simulink model "untitled"  (R2021a)
settings: Solver=FixedStepDiscrete  StartTime=0.0  StopTime=inf  FixedStep=0.1  RelTol=1e-3
settings Model: SILPILModeSetting=veronly  EnablePacing=on  ExtModeTrigDuration=2  Creator=smrh1  LastModifiedBy=Abbas
settings SolverCC: AlgebraicLoopSolver=TrustRegion  AutoInsertRateTranBlk=on
settings OptimizationCC: EnhancedBackFolding=on  PassReuseOutputArgsAs=Individual arguments  ZeroExternalMemoryAtStartup=off  ZeroInternalMemoryAtStartup=off  MaxStackSize=64  OptimizeBlockOrder=speed  DifferentSizesBufferReuse=on  OptimizationCustomize=off  EfficientTunableParamExpr=on
settings DebuggingCC: ParameterTunabilityLossMsg=error  SFUnexpectedBacktrackingDiag=warning  SFNoUnconditionalDefaultTransitionDiag=warning  SFExecutionAtInitializationDiag=none  ArithmeticOperatorsInVariantConditions=warning
settings HardwareCC: ProdBitPerInt=16  ProdBitPerPointer=16  ProdBitPerSizeT=16  ProdBitPerPtrDiffT=16  ProdLargestAtomicFloat=None  ProdWordSize=8  ProdHWDeviceType=Atmel->AVR
settings SFSimCC: SimUseLocalCustomCode=off  MATLABDynamicMemAlloc=off  CustomCodeUndefinedFunction=UseInterfaceOnly
settings RTWCC: SystemTargetFile=ert.tlc  HardwareBoard=Arduino Uno  TemplateMakefile=ert_default_tmf  RTWUseLocalCustomCode=off  Toolchain=Arduino AVR  BuildConfiguration=Faster Runs
settings CodeAppCC: ForceParamTrailComments=on  IgnoreCustomStorageClasses=off  OperatorAnnotations=on  SimulinkDataObjDesc=on  SFDataObjDesc=on  InsertBlockDesc=on
settings ERTTargetCC: SupportContinuousTime=on  SupportVariableSizeSignals=on  ExtModeStaticAllocSize=250
settings ConfigComp: CovMetricSettings=dw  CovSaveCumulativeToWorkspaceVar=on  CovSaveSingleToWorkspaceVar=on  CovExternalEMLEnable=off

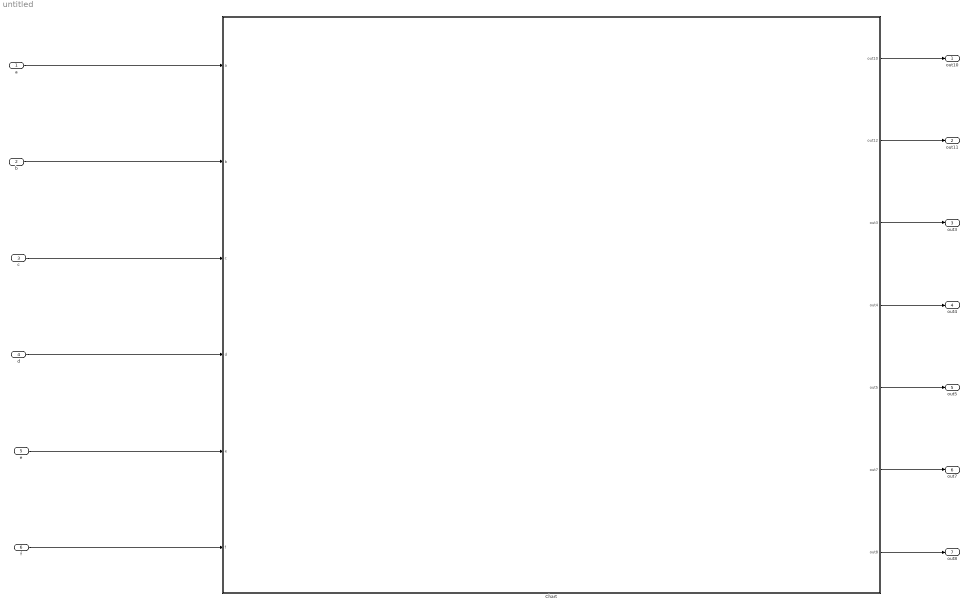
== system untitled ==
  a : Inport
  b : Inport  Port=2
  c : Inport  Port=3
  d : Inport  Port=4
  e : Inport  Port=5
  f : Inport  Port=6
  Chart : Stateflow chart  TreatAsAtomicUnit=on
  out10 : Outport
  out11 : Outport  Port=2
  out3 : Outport  Port=3
  out4 : Outport  Port=4
  out5 : Outport  Port=5
  out7 : Outport  Port=6
  out8 : Outport  Port=7
  wires:
  a/1 -> Chart/1(a)
  b/1 -> Chart/2(b)
  c/1 -> Chart/3(c)
  d/1 -> Chart/4(d)
  e/1 -> Chart/5(e)
  f/1 -> Chart/6(f)
  Chart/1(out10) -> out10/1
  Chart/2(out12) -> out11/1
  Chart/3(out3) -> out3/1
  Chart/4(out4) -> out4/1
  Chart/6(out7) -> out7/1
  Chart/7(out8) -> out8/1
  Chart/5(out5) -> out5/1

== stateflow chart untitled/Chart ==
  state state2
    state state6
      state d [parallel]
        settings: executionOrder=3
        state state8
          entry:
          out8=1;
          during:
          out8 = 1;
          exit:
          out8 = 0;
        state state9
        state9 -> state8 : [a==1]
        state8 -> state9 : [b==1]
        (default) -> state9
      state e [parallel]
        settings: executionOrder=1
        state state10
          entry:
          out10=1;
          during:
          out10 = 1;
          exit:
          out10 = 0;
        state state11
        state11 -> state10 : [c==1]
        state10 -> state11 : [c==1]
        (default) -> state11
      state f [parallel]
        settings: executionOrder=2
        state state12
          entry:
          out12=1;
          during:
          out12 = 1;
          exit:
          out12 = 0;
        state state13
        state13 -> state12 : [c==1]
        state12 -> state13 : [a==1]
        (default) -> state13
    state state7
      entry:
      out7=1;
      during:
      out7 = 1;
      exit:
      out7 = 0;
    state7 -> state6 [order 2] : [e==1]
    state6 -> state7 : [d==1]
    (default) -> state6
  state state1
    (history)
    state state4
      entry:
      out4=1;
      during:
      out4 = 1;
      exit:
      out4 = 0;
    state state5
      entry:
      out5=1;
      during:
      out5 = 1;
      exit:
      out5 = 0;
    (default) -> state4 : {out4 =1}
    state5 -> state4 : [a==1]
    state4 -> state5 : [b==1]
  state state3
    entry:
    out3=1;
    during:
    out3 = 1;
    exit:
    out3 = 0;
  (default) -> state1
  state1 -> state2 [order 1] : [f==1]
  state7 -> state1 [order 1] : [b==1]
  state3 -> state5 : [e==1]
  state1 -> state3 [order 2] : [d==1]
  data: a input; b input; c input; d input; e input; f input; out10 output double; out12 output double; out3 output double; out4 output double; out5 output double; out7 output double; out8 output double
